simulink model "IO301simplepwmcap"  (Simulink 7.4)
settings: Solver=FixedStepDiscrete  StartTime=0.0  StopTime=inf  RelTol=1e-3
PreLoadFcn:
  | fpga_freq = 33e6;
  | Ts = 0.001;
  | Tpwm = 10e-6;
libraries: speedgoatlib_IO301 x3, simulink x2, xpclib x1
settings Model: Creator=dkuratli  LastModifiedBy=lab3  BufferReuse=off
settings OptimizationCC: BlockReduction=off  OptimizeBlockIOStorage=off  BufferReuse=off  ExpressionFolding=off  ExpressionDepthLimit=128  LocalBlockOutputs=off
settings DebuggingCC: UnderspecifiedInitializationDetection=Simplified  FcnCallInpInsideContextMsg=Enable All  StateNameClashWarn=none  StrictBusMsg=ErrorLevel1
settings HardwareCC: ProdIntDivRoundTo=Zero  ProdEndianess=LittleEndian  ProdHWDeviceType=Generic->32-bit x86 compatible
settings RTWCC: SystemTargetFile=xpctarget.tlc  TemplateMakefile=xpc_default_tmf  Description=Simulink Real-Time  RTWVerbose=off  ProcessScript=xpctarget_make_rtw_hook  RTWCompilerOptimization=On
settings CodeAppCC: CustomSymbolStrType=$N$R$M_T
settings xpcTargetCC: TargetFcnLib=ansi_tfl_table_tmw.mat  TargetFunctionLibrary=ANSI_C  ParMdlRefBuildCompliant=on  ConcurrentExecutionCompliant=on  CombineSignalStateStructs=off  GRTInterface=on  GenerateAllocFcn=off  xPCTaskExecutionProfile=off  xPCRL32EventNumber=5000  xPCLoadParamSetFile=off  xPCConcurrentTasks=off  xPCEnableSFAnimation=off

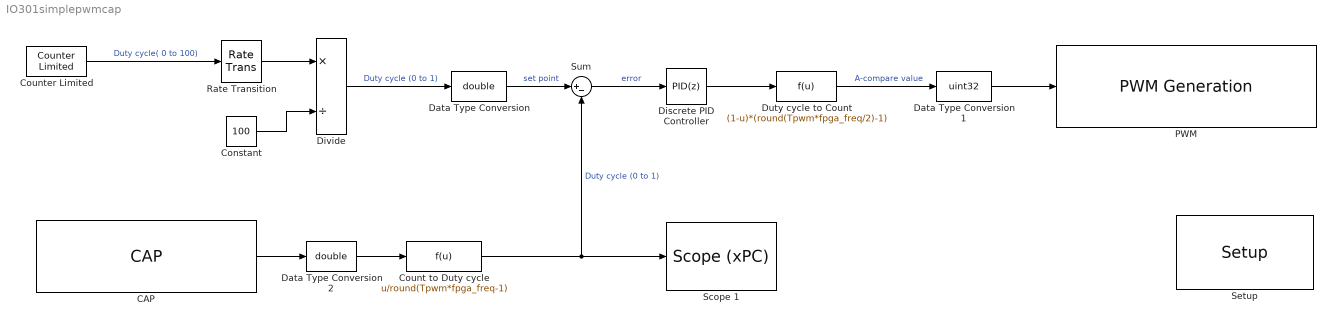
== system IO301simplepwmcap ==
  CAP : speedgoatlib_IO301/CAP/CAP  id=1  channel=[1]  startEvent=[1]  stopEvent=[0]  period=[0]  ts=Ts  pciSlot=-1
  Constant : Constant  Value=100  SampleTime=Ts
  Count to Duty cycle : Fcn  Expr=u/round(Tpwm*fpga_freq-1)
  Counter Limited : simulink/Sources/Counter Limited  uplimit=100  tsamp=0.02
  Data Type Conversion : DataTypeConversion  OutDataTypeStr=double  OutDataTypeMode=double
  Data Type Conversion1 : DataTypeConversion  OutDataTypeStr=uint32  OutDataTypeMode=uint32
  Data Type Conversion2 : DataTypeConversion  OutDataTypeStr=double  OutDataTypeMode=double
  Discrete PID Controller : simulink/Continuous/PID Controller  Controller=PID  TimeDomain=Discrete-time  SampleTime=-1  IntegratorMethod=Forward Euler  FilterMethod=Forward Euler  Form=Parallel  P=0.158384304316701  I=316.768608633401  D=0  N=100  InitialConditionSource=internal  InitialConditionForIntegrator=0  InitialConditionForFilter=0  ExternalReset=none  LimitOutput=off  UpperSaturationLimit=inf  LowerSaturationLimit=-inf  LinearizeAsGain=off  AntiWindupMode=none  Kb=1  TrackingMode=off  Kt=1  PParamMin=[]  PParamMax=[]  IParamMin=[]  IParamMax=[]  DParamMin=[]  DParamMax=[]  NParamMin=[]  NParamMax=[]  KbParamMin=[]  KbParamMax=[]  KtParamMin=[]  KtParamMax=[]  POutMin=[]  POutMax=[]  IOutMin=[]  IOutMax=[]  DOutMin=[]  DOutMax=[]  NOutMin=[]  NOutMax=[]  KbOutMin=[]  KbOutMax=[]  KtOutMin=[]  KtOutMax=[]  IntegratorOutMin=[]  IntegratorOutMax=[]  FilterOutMin=[]  FilterOutMax=[]  SumOutMin=[]  SumOutMax=[]  SumI1OutMin=[]  SumI1OutMax=[]  SumI2OutMin=[]  SumI2OutMax=[]  SumI3OutMin=[]  SumI3OutMax=[]  SumDOutMin=[]  SumDOutMax=[]  SaturationOutMin=[]  SaturationOutMax=[]  IntegratorContinuousStateAttributes=''  IntegratorStateMustResolveToSignalObject=off  IntegratorRTWStateStorageClass=Auto  FilterContinuousStateAttributes=''  FilterStateMustResolveToSignalObject=off  FilterRTWStateStorageClass=Auto
  Divide : Product  Inputs=*/  SampleTime=Ts
  Duty cycle to Count : Fcn  Expr=(1-u)*(round(Tpwm*fpga_freq/2)-1)
  PWM : speedgoatlib_IO301/PWM Generation/PWM Generation  channel=[1]  group=Module setup  id=1  ts=-1  pciSlot=-1  initStart=[1]  toggleAStart=[0]  toggleAStop=[0]  toggleBStart=[1]  toggleBStop=[0]  showStart=off  showAStart=off  showAStop=off  showBStart=off  showBStop=off  initA=[1]  initB=[1]  initC=[round(fpga_freq*Tpwm/2)-1]  showA=on  showB=off  showC=off  initActionA=[0,0,2,1]'  initActionB=[0,0,2,1]'  showActionA=off  showActionB=off  triggerSource=[1]  triggerPulseLength=32  protection=[0]
  Rate Transition : RateTransition
  Scope 1 : xpclib/Misc./Scope (xPC)   scopeno=1  scopetype=Target  autostart=on  viewmode=Graphical redraw  formatstr='%15.6f'  grid=on  ylimits=[0,0]  nosamples=4000  noprepostsamples=0  interleave=1  triggermode=FreeRun  triggersignal=1  trigsignalfromport=off  triggerlevel=0.0  triggerslope=Either  triggerscope=1  triggersample=0  filename=data.dat  mode=Lazy  writesize=512  autorestart=off  dynamicfilemode=off  maxwritefilesize=512*1024^2
  Setup : speedgoatlib_IO301/Setup/Setup  group=Module setup  id=1  fpga1=speedgoat_IO301_default  pciSlot=-1  lowerDirection=[1, 1, 1, 1, 1, 0, 0, 0, 0, 0, 0, 0, 1, 1, 1, 1]  lowerReset=[1]  lowerValue=[0]  upperDirection=[1, 1, 1, 1, 1, 1, 1, 1, 0, 0, 0, 0, 0, 0, 0, 0]  upperReset=[1]  upperValue=[0]
  Sum : Sum  Inputs=|+-
  wires:
  Duty cycle to Count/1 -> Data Type Conversion1/1  "A-compare value"
  Data Type Conversion1/1 -> PWM/1
  CAP/1 -> Data Type Conversion2/1
  Data Type Conversion2/1 -> Count to Duty cycle/1
  Counter Limited/1 -> Rate Transition/1  "Duty cycle( 0 to 100)"
  Divide/1 -> Data Type Conversion/1  "Duty cycle (0 to 1)"
  Count to Duty cycle/1 -> Scope 1/1, Sum/2  "Duty cycle (0 to 1)"
  Constant/1 -> Divide/2
  Data Type Conversion/1 -> Sum/1  "set point"
  Sum/1 -> Discrete PID Controller/1  "error"
  Discrete PID Controller/1 -> Duty cycle to Count/1
  Rate Transition/1 -> Divide/1
